simulink model "NonLinearPlant"  (Simulink 8.2)
settings: Solver=ode4  SolverMode=SingleTasking  StartTime=0.0  StopTime=Tend  FixedStep=h  RelTol=1e-3
values from neighbouring files (symbols this model uses):
  dU = 0    [Analysis_of_a_Nonlinear_Electromechanical_Plant.m]
  J = 0.5e-5    (= 5e-06)    [Analysis_of_a_Nonlinear_Electromechanical_Plant.m]
  Ke = 0.05    [Analysis_of_a_Nonlinear_Electromechanical_Plant.m]
  Km = Ke    (= 0.05)    [Analysis_of_a_Nonlinear_Electromechanical_Plant.m]
  Kpc = 3    [Analysis_of_a_Nonlinear_Electromechanical_Plant.m]
  Kvf = 0.00000    (= 0)    [Analysis_of_a_Nonlinear_Electromechanical_Plant.m]
  M_L = 0.0    (= 0)    [Analysis_of_a_Nonlinear_Electromechanical_Plant.m]
  Mdf = 0.000    (= 0)    [Analysis_of_a_Nonlinear_Electromechanical_Plant.m]
  Ra = 10    [Analysis_of_a_Nonlinear_Electromechanical_Plant.m]
  t_L = Tend/2    (= 0.75)    [Analysis_of_a_Nonlinear_Electromechanical_Plant.m]
  Ta = La/Ra    (= 0.01)    [Analysis_of_a_Nonlinear_Electromechanical_Plant.m]
  Tpc = 0.001    [Analysis_of_a_Nonlinear_Electromechanical_Plant.m]
settings Model: Creator=RIS  LastModifiedBy=RIS
settings DataIOCC: SignalLoggingSaveFormat=Dataset
settings OptimizationCC: ExpressionDepthLimit=128
settings DebuggingCC: FcnCallInpInsideContextMsg=EnableAllAsError  StateNameClashWarn=none
settings GRTTargetCC: CombineOutputUpdateFcns=on  GRTInterface=off

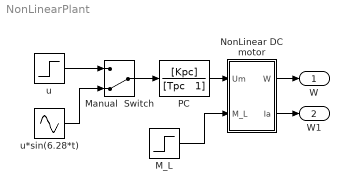
== system NonLinearPlant ==
  " NonLinear DC motor" : Subsystem
  M_L : Step  Time=t_L  After=M_L  SampleTime=0
  Manual  Switch : ManualSwitch  CurrentSetting=0
  PC : TransferFcn  Numerator=[Kpc]  Denominator="[Tpc   1]"
  u : Step  Time=0  After=u  SampleTime=0
  u*sin(6.28*t) : Sin  Amplitude=u  Frequency=6.28  SampleTime=0
  W : Outport
  W1 : Outport  Port=2
  wires:
  " NonLinear DC motor"/1(W) -> W/1
  " NonLinear DC motor"/2(Ia) -> W1/1
  u/1 -> Manual  Switch/1
  u*sin(6.28*t)/1 -> Manual  Switch/2
  Manual  Switch/1 -> PC/1
  PC/1 -> " NonLinear DC motor"/1("Um ")
  M_L/1 -> " NonLinear DC motor"/2(M_L)

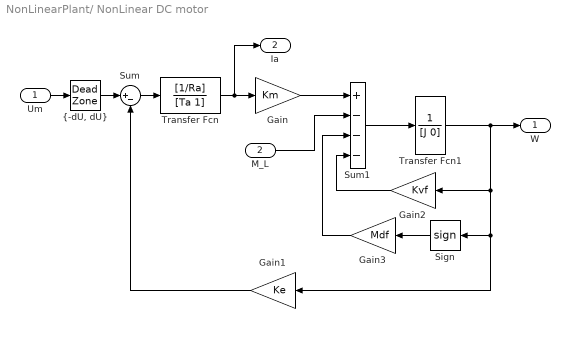
== system NonLinearPlant/ NonLinear DC motor ==
  "Um " : Inport
  M_L : Inport  Port=2
  Gain : Gain  Gain=Km
  Gain1 : Gain  Gain=Ke
  Gain2 : Gain  Gain=Kvf
  Gain3 : Gain  Gain=Mdf
  Sign : Signum
  Sum : Sum  Inputs=|+-
  Sum1 : Sum  Inputs=+---
  Transfer Fcn : TransferFcn  Numerator=[1/Ra]  Denominator=[Ta 1]
  Transfer Fcn1 : TransferFcn  Denominator=[J 0]
  "{-dU, dU}" : DeadZone  LowerValue=-dU  UpperValue=dU  SaturateOnIntegerOverflow=on
  W : Outport
  Ia : Outport  Port=2
  wires:
  Sum/1 -> Transfer Fcn/1
  Transfer Fcn/1 -> Gain/1, Ia/1
  Gain/1 -> Sum1/1
  Sum1/1 -> Transfer Fcn1/1
  Gain1/1 -> Sum/2
  M_L/1 -> Sum1/2
  "Um "/1 -> "{-dU, dU}"/1
  "{-dU, dU}"/1 -> Sum/1
  Gain2/1 -> Sum1/4
  Transfer Fcn1/1 -> Gain2/1, Gain1/1, Sign/1, W/1
  Sign/1 -> Gain3/1
  Gain3/1 -> Sum1/3
